simulink model "QuarterCarModel"  (R2018b)
settings: Solver=VariableStepAuto  StartTime=0.0  StopTime=5  RelTol=1e-3
values from neighbouring files (symbols this model uses):
  cs_c = 15000    [half_parameters.m]    (also in parameters.m = 1000)
  cs_e = cs_c    (= 15000)    [half_parameters.m]    (also in parameters.m = 1000)
  g = 9.81    [half_parameters.m]    (also in parameters.m)
  ks = 15e4    (= 150000)    [half_parameters.m]    (also in parameters.m = 20000)
  ktc = 35e4    (= 350000)    [half_parameters.m]    (also in parameters.m = 140000)
  kte = ktc    (= 350000)    [half_parameters.m]    (also in parameters.m = 140000)
  m1 = 2600    [half_parameters.m]    (also in parameters.m = 250)
  m2 = 20    [half_parameters.m]    (also in parameters.m)
  x0 = 0.2    [half_parameters.m]    (also in parameters.m)
undefined symbols (not defined in the file or in its folder): kstiff
libraries: simulink x1
settings Model: Creator=Hannah  LastModifiedBy=Hannah

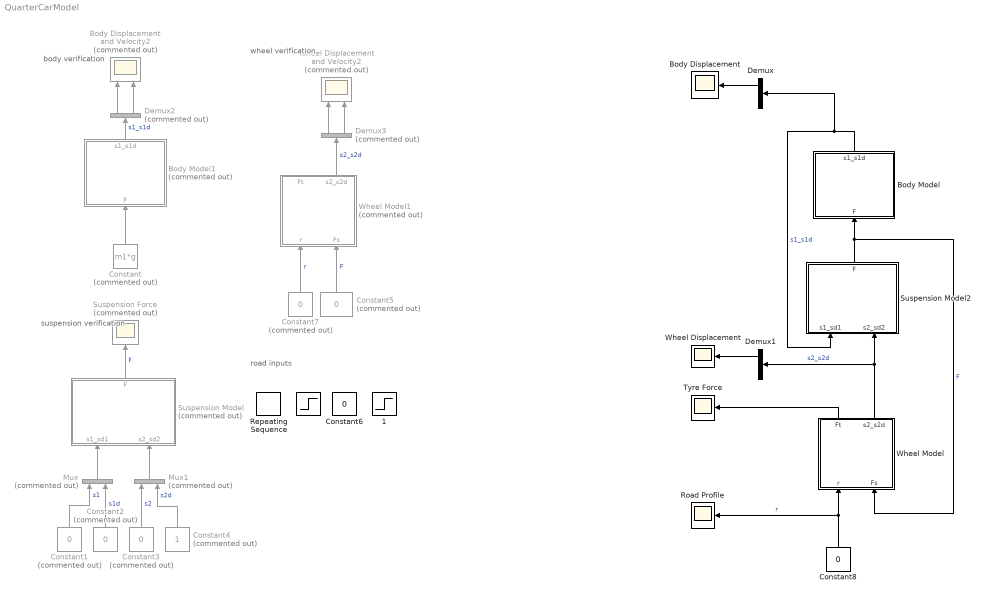
== system QuarterCarModel ==
  note: wheel
      | verification
  note: body
      | verification
  note: suspension
      | verification
  note: road inputs
  " " : Step  SampleTime=0
  " 1" : Step  After=-1  SampleTime=0
  "Body Displacement " : Scope
  Body Displacement and Velocity2 : Scope  Commented=on  NumInputPorts=2
  Body Model : Subsystem
      mask Display: image('body.png')
  Body Model1 : Subsystem  Commented=on
      mask Display: image('body.png')
  Constant : Constant  Commented=on  Value=m1*g
  Constant{1..3,5,7} (5 alike) : Constant  Commented=on  Value=0
  Constant4 : Constant  Commented=on
  Constant6 : Constant  Value=0
  Constant8 : Constant  Value=0
  Demux : Demux  Outputs=2
  Demux1 : Demux  Outputs=2
  Demux2 : Demux  Commented=on  Outputs=2
  Demux3 : Demux  Commented=on  Outputs=2
  Mux : Mux  Commented=on  Inputs=2
  Mux1 : Mux  Commented=on  Inputs=2
  Repeating Sequence : simulink/Sources/Repeating Sequence  rep_seq_t=[0 3 5 10 12 15]  rep_seq_y=[0 0 1 1 0 0]
  Road Profile : Scope
  Suspension Model : Subsystem  Commented=on
      mask Display: image('suspension.png')
  Suspension Model2 : Subsystem
      mask Display: image('suspension.png')
  Suspension Force : Scope  Commented=on
  Tyre Force : Scope
  Wheel Model : Subsystem
      mask Display: image('wheel.png')
  Wheel Model1 : Subsystem  Commented=on
      mask Display: image('wheel.png')
  "Wheel Displacement " : Scope
  Wheel Displacement and Velocity2 : Scope  Commented=on  NumInputPorts=2
  wires:
  Body Model/1(s1_s1d) -> Suspension Model2/1(s1_sd1), Demux/1  "s1_s1d"
  Suspension Model2/1(F) -> Wheel Model/2(Fs), Body Model/1(F)  "F"
  Wheel Model/2(s2_s2d) -> Suspension Model2/2(s2_sd2), Demux1/1  "s2_s2d"
  Demux/1 -> "Body Displacement "/1
  Demux1/1 -> "Wheel Displacement "/1
  Wheel Model/1(Ft) -> Tyre Force/1
  Constant8/1 -> Wheel Model/1(r), Road Profile/1  "r"
  Demux2/1 -> Body Displacement and Velocity2/1
  Body Model1/1(s1_s1d) -> Demux2/1  "s1_s1d"
  Constant/1 -> Body Model1/1(F)
  Demux2/2 -> Body Displacement and Velocity2/2
  Constant1/1 -> Mux/1  "s1"
  Constant2/1 -> Mux/2  "s1d"
  Constant3/1 -> Mux1/1  "s2"
  Constant4/1 -> Mux1/2  "s2d"
  Mux1/1 -> Suspension Model/2(s2_sd2)
  Mux/1 -> Suspension Model/1(s1_sd1)
  Suspension Model/1(F) -> Suspension Force/1  "F"
  Wheel Model1/2(s2_s2d) -> Demux3/1  "s2_s2d"
  Demux3/1 -> Wheel Displacement and Velocity2/1
  Demux3/2 -> Wheel Displacement and Velocity2/2
  Constant5/1 -> Wheel Model1/2(Fs)  "F"
  Constant7/1 -> Wheel Model1/1(r)  "r"

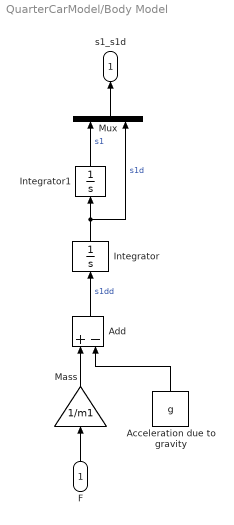
== system QuarterCarModel/Body Model ==
  F : Inport
  "Acceleration due to gravity " : Constant  Value=g
  Add : Sum  Inputs=+-
  Integrator : Integrator
  Integrator1 : Integrator
  Mass : Gain  Gain=1/m1
  Mux : Mux  Inputs=2
  s1_s1d : Outport
  wires:
  Mux/1 -> s1_s1d/1
  Mass/1 -> Add/1
  Integrator/1 -> Mux/2, Integrator1/1  "s1d"
  "Acceleration due to gravity "/1 -> Add/2
  F/1 -> Mass/1
  Integrator1/1 -> Mux/1  "s1"
  Add/1 -> Integrator/1  "s1dd"

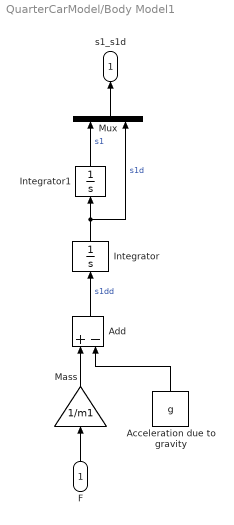
== system QuarterCarModel/Body Model1 ==
  F : Inport
  "Acceleration due to gravity " : Constant  Value=g
  Add : Sum  Inputs=+-
  Integrator : Integrator
  Integrator1 : Integrator
  Mass : Gain  Gain=1/m1
  Mux : Mux  Inputs=2
  s1_s1d : Outport
  wires:
  Mux/1 -> s1_s1d/1
  Mass/1 -> Add/1
  Integrator/1 -> Mux/2, Integrator1/1  "s1d"
  "Acceleration due to gravity "/1 -> Add/2
  F/1 -> Mass/1
  Integrator1/1 -> Mux/1  "s1"
  Add/1 -> Integrator/1  "s1dd"

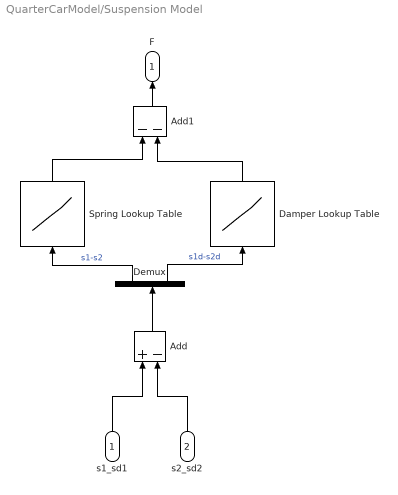
== system QuarterCarModel/Suspension Model ==
  s1_sd1 : Inport
  s2_sd2 : Inport  Port=2
  Add : Sum  Inputs=+-
  Add1 : Sum  Inputs=--
  Damper Lookup Table : Lookup_n-D  NumberOfTableDimensions=1  BreakpointsForDimension1=[-1 0 1]  Table=[-cs_c, 0, cs_e]  InternalRulePriority=Speed  RndMeth=Simplest  InputSameDT=on
  Demux : Demux  Outputs=2
  Spring Lookup Table : Lookup_n-D  NumberOfTableDimensions=1  BreakpointsForDimension1=[-2*x0, -x0, x0, 2*x0]  Table=[-(ks+kstiff)*x0, -ks*x0, ks*x0, (ks+kstiff)*x0]  InternalRulePriority=Speed  RndMeth=Simplest  InputSameDT=on
  F : Outport
  wires:
  s2_sd2/1 -> Add/2
  Spring Lookup Table/1 -> Add1/1
  Add1/1 -> F/1
  Damper Lookup Table/1 -> Add1/2
  Demux/2 -> Damper Lookup Table/1  "s1d-s2d"
  Demux/1 -> Spring Lookup Table/1  "s1-s2"
  Add/1 -> Demux/1
  s1_sd1/1 -> Add/1

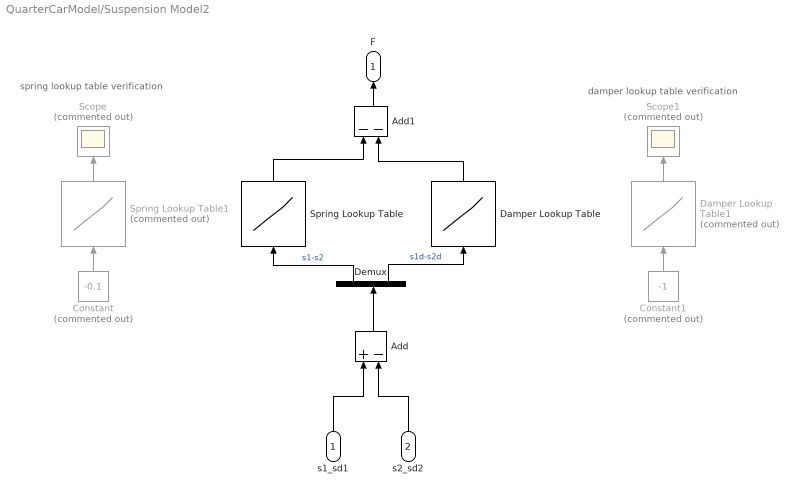
== system QuarterCarModel/Suspension Model2 ==
  note: spring lookup table verification
  note: damper lookup table verification
  s1_sd1 : Inport
  s2_sd2 : Inport  Port=2
  Add : Sum  Inputs=+-
  Add1 : Sum  Inputs=--
  Constant : Constant  Commented=on  Value=-0.1
  Constant1 : Constant  Commented=on  Value=-1
  Damper Lookup Table : Lookup_n-D  NumberOfTableDimensions=1  BreakpointsForDimension1=[-1 0 1]  Table=[-cs_c, 0, cs_e]  InternalRulePriority=Speed  RndMeth=Simplest  InputSameDT=on
  Damper Lookup Table1 : Lookup_n-D  Commented=on  NumberOfTableDimensions=1  BreakpointsForDimension1=[-1 0 1]  Table=[-cs_c, 0, cs_e]  InternalRulePriority=Speed  RndMeth=Simplest  InputSameDT=on
  Demux : Demux  Outputs=2
  Scope : Scope  Commented=on
  Scope1 : Scope  Commented=on
  Spring Lookup Table : Lookup_n-D  NumberOfTableDimensions=1  BreakpointsForDimension1=[-2*x0, -x0, x0, 2*x0]  Table=[-(ks+kstiff)*x0, -ks*x0, ks*x0, (ks+kstiff)*x0]  InternalRulePriority=Speed  RndMeth=Simplest  InputSameDT=on
  Spring Lookup Table1 : Lookup_n-D  Commented=on  NumberOfTableDimensions=1  BreakpointsForDimension1=[-2*x0, -x0, x0, 2*x0]  Table=[-(ks+kstiff)*x0, -ks*x0, ks*x0, (ks+kstiff)*x0]  InternalRulePriority=Speed  RndMeth=Simplest  InputSameDT=on
  F : Outport
  wires:
  s2_sd2/1 -> Add/2
  Spring Lookup Table/1 -> Add1/1
  Add1/1 -> F/1
  Damper Lookup Table/1 -> Add1/2
  Demux/2 -> Damper Lookup Table/1  "s1d-s2d"
  Demux/1 -> Spring Lookup Table/1  "s1-s2"
  Add/1 -> Demux/1
  s1_sd1/1 -> Add/1
  Constant/1 -> Spring Lookup Table1/1
  Constant1/1 -> Damper Lookup Table1/1
  Spring Lookup Table1/1 -> Scope/1
  Damper Lookup Table1/1 -> Scope1/1

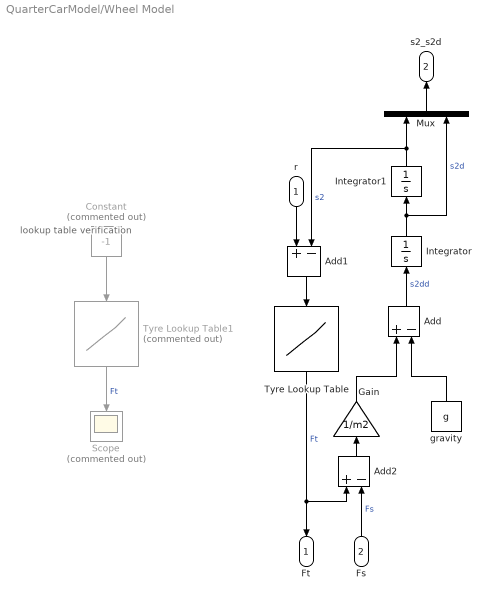
== system QuarterCarModel/Wheel Model ==
  note: lookup table
      | verification
  r : Inport
  Fs : Inport  Port=2
  Add : Sum  Inputs=+-
  Add1 : Sum  Inputs=+-
  Add2 : Sum  Inputs=+-
  Constant : Constant  Commented=on  Value=-1
  Gain : Gain  Gain=1/m2
  Integrator : Integrator
  Integrator1 : Integrator
  Mux : Mux  Inputs=2
  Scope : Scope  Commented=on
  Tyre Lookup Table : Lookup_n-D  NumberOfTableDimensions=1  BreakpointsForDimension1=[-1 0 1]  Table=[-kte, 0, ktc]  InternalRulePriority=Speed  RndMeth=Simplest  InputSameDT=on
  Tyre Lookup Table1 : Lookup_n-D  Commented=on  NumberOfTableDimensions=1  BreakpointsForDimension1=[-1 0 1]  Table=[-kte, 0, ktc]  InternalRulePriority=Speed  RndMeth=Simplest  InputSameDT=on
  gravity : Constant  Value=g
  Ft : Outport
  s2_s2d : Outport  Port=2
  wires:
  r/1 -> Add1/1
  Fs/1 -> Add2/2  "Fs"
  Add2/1 -> Gain/1
  Gain/1 -> Add/1
  Integrator/1 -> Mux/2, Integrator1/1  "s2d"
  Add/1 -> Integrator/1  "s2dd"
  Tyre Lookup Table/1 -> Ft/1, Add2/1  "Ft"
  gravity/1 -> Add/2
  Integrator1/1 -> Add1/2, Mux/1  "s2"
  Add1/1 -> Tyre Lookup Table/1
  Mux/1 -> s2_s2d/1
  Constant/1 -> Tyre Lookup Table1/1
  Tyre Lookup Table1/1 -> Scope/1  "Ft"

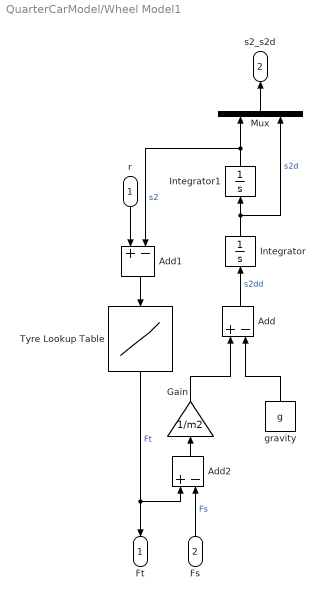
== system QuarterCarModel/Wheel Model1 ==
  r : Inport
  Fs : Inport  Port=2
  Add : Sum  Inputs=+-
  Add1 : Sum  Inputs=+-
  Add2 : Sum  Inputs=+-
  Gain : Gain  Gain=1/m2
  Integrator : Integrator
  Integrator1 : Integrator  InitialCondition=1
  Mux : Mux  Inputs=2
  Tyre Lookup Table : Lookup_n-D  NumberOfTableDimensions=1  BreakpointsForDimension1=[-1 0 1]  Table=[-kte, 0, ktc]  InternalRulePriority=Speed  RndMeth=Simplest  InputSameDT=on
  gravity : Constant  Value=g
  Ft : Outport
  s2_s2d : Outport  Port=2
  wires:
  r/1 -> Add1/1
  Fs/1 -> Add2/2  "Fs"
  Add2/1 -> Gain/1
  Gain/1 -> Add/1
  Integrator/1 -> Mux/2, Integrator1/1  "s2d"
  Add/1 -> Integrator/1  "s2dd"
  Tyre Lookup Table/1 -> Ft/1, Add2/1  "Ft"
  gravity/1 -> Add/2
  Integrator1/1 -> Add1/2, Mux/1  "s2"
  Add1/1 -> Tyre Lookup Table/1
  Mux/1 -> s2_s2d/1
